simulink model "Junctions1_integers"  (R2017b)
settings: Solver=FixedStepDiscrete  StartTime=0.0  StopTime=10.0  FixedStep=0.200000  RelTol=1e-3  EnableMultiTasking=on
model workspace (MAT data in the model file):
  already_pp = 1
settings Model: ExtModeAutoUpdateStatusClock=off  Creator=scaife  LastModifiedBy=hbourbou
settings DataIOCC: LimitDataPoints=on  SaveFormat=Array  SignalLoggingSaveFormat=ModelDataLogs  SignalLoggingName=sigsOut
settings OptimizationCC: LifeSpan=inf
settings DebuggingCC: AlgebraicLoopMsg=error  ArtificialAlgebraicLoopMsg=error  SaveWithParameterizedLinksMsg=none  UnderspecifiedInitializationDetection=Classic  MergeDetectMultiDrivingBlocksExec=none  SignalResolutionControl=TryResolveAllWithWarning  MultiTaskDSMMsg=warning  MultiTaskCondExecSysMsg=none  SingleTaskRateTransMsg=error  SFUnexpectedBacktrackingDiag=warning  SFNoUnconditionalDefaultTransitionDiag=warning  SFExecutionAtInitializationDiag=none
settings HardwareCC: ProdBitPerPointer=32  ProdBitPerSizeT=32  ProdBitPerPtrDiffT=32  ProdLargestAtomicFloat=None  ProdIntDivRoundTo=Undefined  ProdEndianess=Unspecified  ProdWordSize=32  ProdHWDeviceType=32-bit Generic  TargetUnknown=on
settings ModelReferenceCC: PropagateSignalLabelsOutOfModel=off
settings SFSimCC: SimParseCustomCode=off
settings CodeAppCC: StateflowObjectComments=on
settings GRTTargetCC: TargetLangStandard=C89/C90 (ANSI)  GeneratePreprocessorConditionals=Disable all  CombineOutputUpdateFcns=off  GRTInterface=on
settings ConfigComp: CovMetricSettings=dw  CovHtmlReporting=on  CovSaveCumulativeToWorkspaceVar=on  CovSaveSingleToWorkspaceVar=on  CovExternalEMLEnable=off

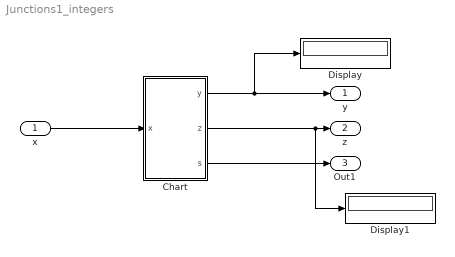
== system Junctions1_integers ==
  x : Inport  OutDataTypeStr=uint32
  Chart : Stateflow chart  TreatAsAtomicUnit=on
  Display : Display
  Display1 : Display
  y : Outport
  z : Outport  Port=2
  Out1 : Outport  Port=3
  wires:
  x/1 -> Chart/1(x)
  Chart/1(y) -> y/1, Display/1
  Chart/2(z) -> Display1/1, z/1
  Chart/3(s) -> Out1/1

== stateflow chart Junctions1_integers/Chart ==
  state A
    ex : y=y/2;
    en: s = 1;
  state C
    ex: y = y+2;
    en: s = 3;
  state B
    ex: y = mod(y,2);
    en: s = 2;
  B -> A : [x>3]
  (default) -> A
  C -> A : [x>3]
  A -> (junction 10) : [x>0]{y = y + 1;z = z + 2}
  (junction 10) -> C [order 2] : [x<2]{y = y + 1;z = z + 1}
  (junction 10) -> B [order 1] : [x>=2]{y = y + 2;z = z + 1}
  data: x input uint32; y output uint32 =uint32(1); z output uint32 =uint32(2); s output uint32
